simulink model "model"  (R2024a)
settings: Solver=FixedStepAuto  StartTime=0.0  StopTime=8  FixedStep=0.0001  RelTol=1e-3
values from neighbouring files (symbols this model uses):
  D = [-3 0; 0 1]    [K.m]    (also in graphs.m; graphs_f.m = 1 - omega.^2 - 1i*omega; graphs_f_log.m = 1 - omega.^2 - 1i*omega)
  L = -Pl*ovC'*inv(R)    [K.m]
  ovA = [Gamma zeros(8, 2); Bf*Y1 A]    [K.m]
  ovB = [zeros(8, 2); B]    [K.m]
  ovC = [Df*Y2-Yg C]    [K.m]
  ovK = [Kwsol Kx]    [K.m]
  w0 = [1; 0; 1; 0; 1; 0; 1; 0]    [K.m]
  x0 = [1; 1]    [K.m]
settings Model: Creator=ventus  LastModifiedBy=ventus

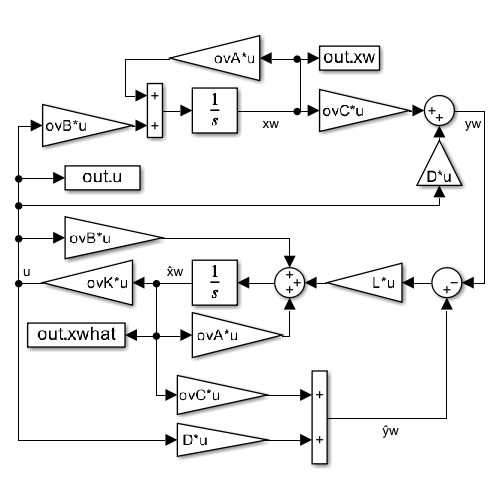
[thumbnail: Simulink's stored preview of the top-level diagram]
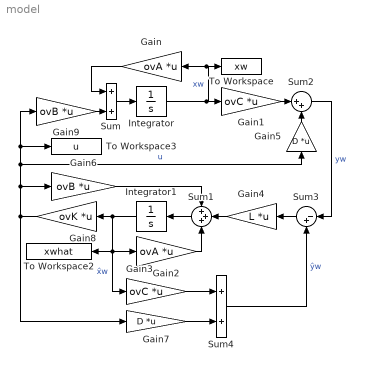
== system model ==
  Gain : Gain  Gain=ovA  Multiplication=Matrix(K*u)
  Gain1 : Gain  Gain=ovC  Multiplication=Matrix(K*u)
  Gain2 : Gain  Gain=ovA  Multiplication=Matrix(K*u)
  Gain3 : Gain  Gain=ovC  Multiplication=Matrix(K*u)
  Gain4 : Gain  Gain=L  Multiplication=Matrix(K*u)
  Gain5 : Gain  Gain=D  Multiplication=Matrix(K*u)
  Gain6 : Gain  Gain=ovB  Multiplication=Matrix(K*u)
  Gain7 : Gain  Gain=D  Multiplication=Matrix(K*u)
  Gain8 : Gain  Gain=ovK  Multiplication=Matrix(K*u)
  Gain9 : Gain  Gain=ovB  Multiplication=Matrix(K*u)
  Integrator : Integrator  InitialCondition=[w0; x0]
  Integrator1 : Integrator  InitialCondition=[0; 0; 0; 0; 0; 0; 0; 0; 0; 0]
  Sum : Sum
  Sum1 : Sum  Inputs=+++
  Sum2 : Sum  Inputs=|++
  Sum3 : Sum  Inputs=|-+
  Sum4 : Sum
  To Workspace : ToWorkspace  VariableName=xw  SaveFormat=Timeseries  SampleTime=-1
  To Workspace2 : ToWorkspace  VariableName=xwhat  SaveFormat=Timeseries  SampleTime=-1
  To Workspace3 : ToWorkspace  VariableName=u  SaveFormat=Timeseries  SampleTime=-1
  wires:
  Gain4/1 -> Sum1/2
  Sum3/1 -> Gain4/1
  Gain/1 -> Sum/1
  Integrator1/1 -> Gain2/1, Gain3/1, To Workspace2/1, Gain8/1  "x̂w"
  Sum2/1 -> Sum3/1  "yw"
  Sum1/1 -> Integrator1/1
  Gain2/1 -> Sum1/3
  Sum/1 -> Integrator/1
  Integrator/1 -> Gain/1, To Workspace/1, Gain1/1  "xw"
  Gain1/1 -> Sum2/1
  Gain8/1 -> Gain5/1, To Workspace3/1, Gain9/1, Gain6/1, Gain7/1  "u"
  Gain9/1 -> Sum/2
  Gain6/1 -> Sum1/1
  Gain5/1 -> Sum2/2
  Sum4/1 -> Sum3/2  "ŷw"
  Gain7/1 -> Sum4/2
  Gain3/1 -> Sum4/1
